simulink model "pulse_detector_v3"  (R2019a)
settings: Solver=FixedStepDiscrete  StartTime=0.0  StopTime=SimTime  RelTol=1e-3
undefined symbols (not defined in the file): CorrFilter, RxSignal, threshold, WindowLen
libraries: dspsrcs4 x2, simulink x1, hdlsllib x1
settings Model: DataTypeOverride=Off  Creator=cchung  LastModifiedBy=cchung
settings DataIOCC: SaveOutput=off  SaveTime=off
settings OptimizationCC: BlockReduction=off  ConditionallyExecuteInputs=off  DefaultParameterBehavior=Inlined
settings DebuggingCC: AlgebraicLoopMsg=error  SingleTaskRateTransMsg=error  PregeneratedLibrarySubsystemCodeDiagnostic=none  ArithmeticOperatorsInVariantConditions=warning
settings HardwareCC: ProdBitPerPointer=32  ProdBitPerSizeT=32  ProdBitPerPtrDiffT=32  ProdLargestAtomicFloat=None  ProdIntDivRoundTo=Undefined  ProdEndianess=Unspecified  ProdWordSize=32  ProdHWDeviceType=ASIC/FPGA->ASIC/FPGA  TargetBitPerPointer=64  TargetBitPerSizeT=64  TargetBitPerPtrDiffT=64  TargetLongLongMode=on  TargetIntDivRoundTo=Zero  TargetEndianess=LittleEndian  TargetWordSize=64  TargetHWDeviceType=Custom Processor->MATLAB Host Computer  ProdEqTarget=off
settings SFSimCC: SimUseLocalCustomCode=off
settings RTWCC: RTWUseLocalCustomCode=off

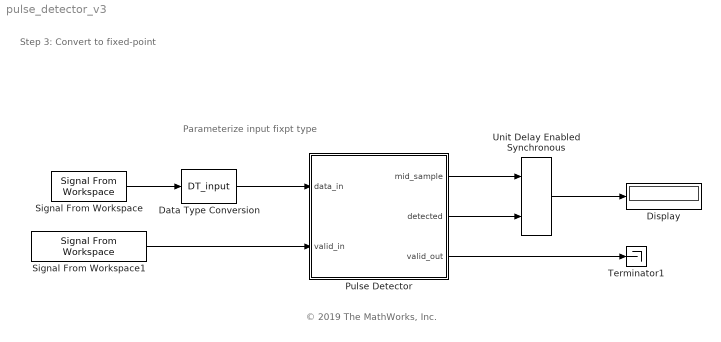
== system pulse_detector_v3 ==
  note: Parameterize input fixpt type
  note: Step 3: Convert to fixed-point
  note: © 2019 The MathWorks, Inc.
  Data Type Conversion : DataTypeConversion  OutDataTypeStr=DT_input  RndMeth=Nearest  SaturateOnIntegerOverflow=on
  Display : Display
  Pulse Detector : Subsystem
  Signal From Workspace : dspsrcs4/Signal From Workspace  X=RxSignal  Ts=1  nsamps=1  OutputAfterFinalValue=Setting to zero  ignoreOrWarnInputAndFrameLengths=off  OutputFrames=off
  Signal From Workspace1 : dspsrcs4/Signal From Workspace  X=true(size(RxSignal))  Ts=1  nsamps=1  OutputAfterFinalValue=Setting to zero  ignoreOrWarnInputAndFrameLengths=off  OutputFrames=off
  Terminator1 : Terminator
  Unit Delay Enabled Synchronous : hdlsllib/Discrete/Unit Delay Enabled Synchronous  InitialCondition=0.0  SampleTime=-1
      settings: SourceProductName=HDL Coder  SourceProductBaseCode=HD
  wires:
  Pulse Detector/1(mid_sample) -> Unit Delay Enabled Synchronous/1
  Data Type Conversion/1 -> Pulse Detector/1(data_in)
  Signal From Workspace1/1 -> Pulse Detector/2(valid_in)
  Signal From Workspace/1 -> Data Type Conversion/1
  Pulse Detector/3(valid_out) -> Terminator1/1
  Pulse Detector/2(detected) -> Unit Delay Enabled Synchronous/2
  Unit Delay Enabled Synchronous/1 -> Display/1

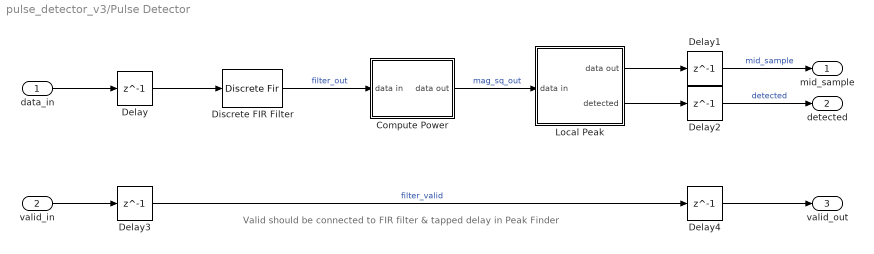
== system pulse_detector_v3/Pulse Detector ==
  note: Valid should be connected to FIR filter & tapped delay in Peak Finder
  data_in : Inport
  valid_in : Inport  Port=2
  Compute Power : Subsystem
      settings: AttributesFormatString=|
      | Architecture : Module
      | AdaptivePipelining : on
      | InputPipeline : 1
      | OutputPipeline : 1
  Delay{,1..4} (5 alike) : Delay  DelayLength=1
  Discrete FIR Filter : DiscreteFir  FilterStructure=Direct form transposed  Coefficients=CorrFilter  CoefDataTypeStr=DT_coeff
      settings: AttributesFormatString=|
      | Architecture : Fully Parallel
      | InputPipeline : 1
      | MultiplierInputPipeline : 1
      | MultiplierOutputPipeline : 1
      | OutputPipeline : 1
  Local Peak : Subsystem
  mid_sample : Outport
  detected : Outport  Port=2
  valid_out : Outport  Port=3
  wires:
  Compute Power/1(data out) -> Local Peak/1(data in)  "mag_sq_out"
  Local Peak/1(data out) -> Delay1/1
  data_in/1 -> Delay/1
  Local Peak/2(detected) -> Delay2/1
  Delay1/1 -> mid_sample/1  "mid_sample"
  Delay2/1 -> detected/1  "detected"
  valid_in/1 -> Delay3/1
  Delay4/1 -> valid_out/1
  Delay/1 -> Discrete FIR Filter/1
  Discrete FIR Filter/1 -> Compute Power/1(data in)  "filter_out"
  Delay3/1 -> Delay4/1  "filter_valid"

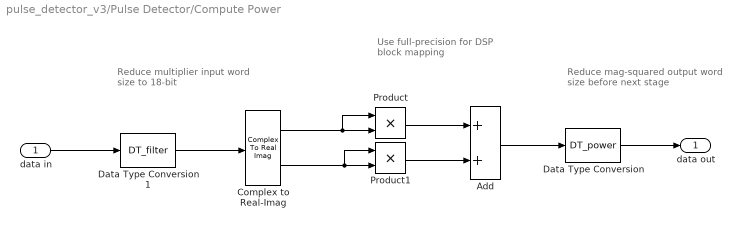
== system pulse_detector_v3/Pulse Detector/Compute Power ==
  note: Use full-precision for
      | DSP block mapping
  note: Reduce mag-squared output
      | word size before next stage
  note: Reduce multiplier input
      | word size to 18-bit
  data in : Inport
  Add : Sum
  Complex to Real-Imag : ComplexToRealImag
  Data Type Conversion : DataTypeConversion  OutDataTypeStr=DT_power
  Data Type Conversion1 : DataTypeConversion  OutDataTypeStr=DT_filter
  Product : Product
  Product1 : Product
  data out : Outport
  wires:
  Complex to Real-Imag/1 -> Product/1, Product/2
  Complex to Real-Imag/2 -> Product1/1, Product1/2
  Product1/1 -> Add/2
  Product/1 -> Add/1
  data in/1 -> Data Type Conversion1/1
  Add/1 -> Data Type Conversion/1
  Data Type Conversion/1 -> data out/1
  Data Type Conversion1/1 -> Complex to Real-Imag/1

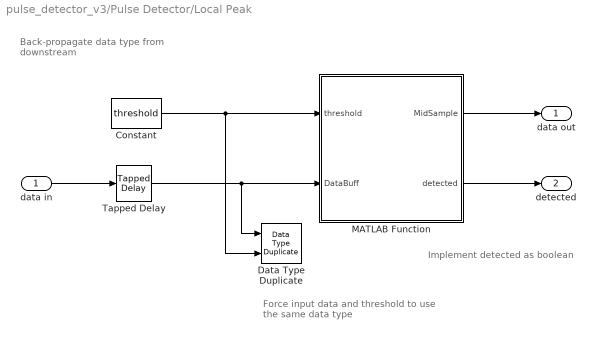
== system pulse_detector_v3/Pulse Detector/Local Peak ==
  note: Force input data and threshold
      | to use the same data type
  note: Implement detected as boolean
  note: Back-propagate data type
      | from downstream
  data in : Inport
  Constant : Constant  Value=threshold  OutDataTypeStr=Inherit: Inherit via back propagation
  Data Type Duplicate : DataTypeDuplicate
  MATLAB Function : MATLAB Function  TreatAsAtomicUnit=on
  Tapped Delay : simulink/Discrete/Tapped Delay  vinit=0.0  samptime=-1  NumDelays=WindowLen  DelayOrder=Oldest  includeCurrent=off
  data out : Outport
  detected : Outport  Port=2
  wires:
  data in/1 -> Tapped Delay/1
  Constant/1 -> Data Type Duplicate/2, MATLAB Function/1(threshold)
  MATLAB Function/1(MidSample) -> data out/1
  MATLAB Function/2(detected) -> detected/1
  Tapped Delay/1 -> Data Type Duplicate/1, MATLAB Function/2(DataBuff)

== matlab function pulse_detector_v3/Pulse Detector/Local Peak/MATLAB Function ==
  data: WindowLen parameter; threshold input; DataBuff input; MidSample output; detected output
function [MidSample,detected] = fcn(WindowLen, threshold, DataBuff)
%#codegen

% Hardware friendly implementation of peak finder
% Modify MATLAB reference as followed:
%
% Define function inputs:
% - WindowLen: non-tunable parameter defined under Simulink->Edit Data
% - threhold: input port (connected to constant)
% - DataBuff: input port (buffering done using Simulink block)
% Define function outputs:
% - Set "detected" when MidSample is local max

MidIdx = ceil(WindowLen/2);

% Compare each value in the window to the middle sample via subtraction
MidSample = DataBuff(MidIdx);
CompareOut = DataBuff - MidSample; % this is a vector

% if all values in the result are negative and the middle sample is
% greater than a threshold, it is a local max
if all(CompareOut <= 0) && (MidSample > threshold)
    detected = true;
else
    detected = false;
end
